simulink model "x2Stage_Rocket"  (R2022b)
settings: Solver=VariableStepAuto  StartTime=0.0  StopTime=5
model workspace: external: MATLAB File C:\Users\Trenton VerKuilen\OneDrive - lmu.edu\School\Capstone\SimscapeImportFiles\x2Stage_Rocket_DataFile.m (data not in the file)
undefined symbols (not defined in the file or in its folder): F, MIL, Moderate, sigbuilder_block, smiData, X, Y, Z
libraries: sm_lib x543, nesl_utility x11, simulink_extras x3, sharedtransform x2, dspmtrx3 x2, aerolibwind2 x2, mspsensorlib x1, aerolibatmos2 x1
(part 11 of 11)

== system x2Stage_Rocket/Model/S1_AvionicsStack_1_RIGID/Stage_2_Electronics_1_RIGID/x2652_BMP280_STEMMA_QT_step_1_RIGID/PCB_Component_step_1_RIGID/x10uF_step_1_RIGID ==
  ReferenceFrame : sm_lib/Frames and Transforms/Reference Frame
  Solid : sm_lib/Body Elements/File Solid  ExtGeomFileName=10uF.step_Default_sldprt.STEP  UnitType=FromFile  ExtGeomFileUnits=m  StepReaderType=HEX  ExportConvexHullGeometry=off  InertiaType=Custom  Mass=smiData.Solid(12).mass  MassUnits=kg  CenterOfMass=smiData.Solid(12).CoM  CenterOfMassUnits=mm  MomentsOfInertia=smiData.Solid(12).MoI  MomentsOfInertiaUnits=kg*mm^2  ProductsOfInertia=smiData.Solid(12).PoI  ProductsOfInertiaUnits=kg*mm^2  BasedOnType=DensityFromFile  Density=1000  DensityUnits=kg/m^3  DoExposeReferenceFrame=on  SerializedFrames=<Frames/>  GraphicType=FromGeometry  MarkerShape=Sphere  MarkerSize=10  GraphicVisPropType=SimpleVisualProperties  GraphicDiffuseColor=smiData.Solid(12).color  GraphicSpecularColor=[0.5 0.5 0.5 1.0]  GraphicAmbientColor=[0.15 0.15 0.15 1.0]  GraphicEmissiveColor=[0.0 0.0 0.0 1.0]  GraphicShininess=75  GraphicOpacity=smiData.Solid(12).opacity
  F : PMIOPort  Side=Left
  connections:
  ReferenceFrame/RConn1 -- Solid/RConn1 -- F/RConn1

== system x2Stage_Rocket/Model/S1_AvionicsStack_1_RIGID/Stage_2_Electronics_1_RIGID/x2652_BMP280_STEMMA_QT_step_1_RIGID/PCB_Component_step_1_RIGID/x10uF_step_2_RIGID ==
  ReferenceFrame : sm_lib/Frames and Transforms/Reference Frame
  Solid : sm_lib/Body Elements/File Solid  ExtGeomFileName=10uF.step_Default_sldprt.STEP  UnitType=FromFile  ExtGeomFileUnits=m  StepReaderType=HEX  ExportConvexHullGeometry=off  InertiaType=Custom  Mass=smiData.Solid(12).mass  MassUnits=kg  CenterOfMass=smiData.Solid(12).CoM  CenterOfMassUnits=mm  MomentsOfInertia=smiData.Solid(12).MoI  MomentsOfInertiaUnits=kg*mm^2  ProductsOfInertia=smiData.Solid(12).PoI  ProductsOfInertiaUnits=kg*mm^2  BasedOnType=DensityFromFile  Density=1000  DensityUnits=kg/m^3  DoExposeReferenceFrame=on  SerializedFrames=<Frames/>  GraphicType=FromGeometry  MarkerShape=Sphere  MarkerSize=10  GraphicVisPropType=SimpleVisualProperties  GraphicDiffuseColor=smiData.Solid(12).color  GraphicSpecularColor=[0.5 0.5 0.5 1.0]  GraphicAmbientColor=[0.15 0.15 0.15 1.0]  GraphicEmissiveColor=[0.0 0.0 0.0 1.0]  GraphicShininess=75  GraphicOpacity=smiData.Solid(12).opacity
  F : PMIOPort  Side=Left
  connections:
  ReferenceFrame/RConn1 -- Solid/RConn1 -- F/RConn1

== system x2Stage_Rocket/Model/S1_AvionicsStack_1_RIGID/Stage_2_Electronics_1_RIGID/x2652_BMP280_STEMMA_QT_step_1_RIGID/PCB_Component_step_1_RIGID/x1N4148_step_1_RIGID ==
  ReferenceFrame : sm_lib/Frames and Transforms/Reference Frame
  Solid : sm_lib/Body Elements/File Solid  ExtGeomFileName=1N4148.step_Default_sldprt.STEP  UnitType=FromFile  ExtGeomFileUnits=m  StepReaderType=HEX  ExportConvexHullGeometry=off  InertiaType=Custom  Mass=smiData.Solid(19).mass  MassUnits=kg  CenterOfMass=smiData.Solid(19).CoM  CenterOfMassUnits=mm  MomentsOfInertia=smiData.Solid(19).MoI  MomentsOfInertiaUnits=kg*mm^2  ProductsOfInertia=smiData.Solid(19).PoI  ProductsOfInertiaUnits=kg*mm^2  BasedOnType=DensityFromFile  Density=1000  DensityUnits=kg/m^3  DoExposeReferenceFrame=on  SerializedFrames=<Frames/>  GraphicType=FromGeometry  MarkerShape=Sphere  MarkerSize=10  GraphicVisPropType=SimpleVisualProperties  GraphicDiffuseColor=smiData.Solid(19).color  GraphicSpecularColor=[0.5 0.5 0.5 1.0]  GraphicAmbientColor=[0.15 0.15 0.15 1.0]  GraphicEmissiveColor=[0.0 0.0 0.0 1.0]  GraphicShininess=75  GraphicOpacity=smiData.Solid(19).opacity
  F : PMIOPort  Side=Left
  connections:
  ReferenceFrame/RConn1 -- Solid/RConn1 -- F/RConn1

== matlab function x2Stage_Rocket/Plant/Aerodynamics/Airframe/Fins Stage 1 ==
  data: C_P_f1 output size=1; C_N_f1 output size=2; C_A_f1 output size=2; AoA input; d_bt input; Re input
function [C_P_f1, C_N_f1, C_A_f1]  = fcn(AoA, d_bt,Re) %only for trapezoidal fins
[C_N_f1, C_P_f1, C_A_f1] = Fins_Stage_1_Coefficients(d_bt, AoA, Re);

== matlab function x2Stage_Rocket/Plant/Overall Rocket/If_on_rail_don't_change ==
  data: Angles input; XYZ_Coords input; Angles_real output; change output
function [Angles_real, change] = fcn(Angles, XYZ_Coords)
[Angles_real, change] = If_on_rail_dont_change(XYZ_Coords, Angles);

== matlab function x2Stage_Rocket/Plant/Overall Rocket/Combine Forces and Convert to Cartesian ==
  data: XYZ_Inertial_Force input; Cart_Accel output; DCM input; Impulse input; Mass input; Inertial_Accel output
function [Cart_Accel,Inertial_Accel]  = fcn(XYZ_Inertial_Force, DCM, Impulse, Mass)
[Cart_Accel,Inertial_Accel] = Combine_Forces_and_Convert_to_Cartesian(XYZ_Inertial_Force, Impulse, Mass, DCM);

== matlab function x2Stage_Rocket/Plant/Aerodynamics/MATLAB Function1 ==
  data: AoA input; Solvable output
function Solvable = fcn(AoA)
if abs(AoA) > deg2rad(15)
    Solvable = 0;
else
    Solvable = 1;
end

== matlab function x2Stage_Rocket/Plant/Aerodynamics/Air Properties/MATLAB Function ==
  settings: updateMethod=CONTINUOUS  sampleTime=0.1
  data: t input; p input; rho output; h input; nu output
function [rho,nu] = AirDensityViscosity(t, p, h)



% AirProperties calculates a variety of air thermodynamic properties from 
% measured values of temperature, pressure and humidity. 
% 
% Variables able to calcuated: 
%   rho         [kg m^-3]       Density
%   mu          [N s m^-2]      Dynamic viscosity
%   k           [W m^-1 K^-1]   Thermal conductivity
%   c_p         [J kg^-1 K^-1]  Specific heat capacity (constant pressure)
%   c_v         [J kg^-1 K^-1]  Specific heat capacity (constant volume)
%   gamma       [1]             Ratio of specific heats
%   c           [m s^-1]        Speed of sound: c = (gamma*R*T/M)^0.5
%   nu          [m^2 s^-1]      Kinematic viscosity: nu = mu/rho
%   alpha       [m^2 s^-1]      Thermal diffusivity: alpha = k/(rho*c_p)
%   Pr          [1]             Prandtl number: Pr = mu*c_p/k
%   M           [kg mol^-1]     Molar mass of humid air
%   R           [J kg^-1 K^-1]  Specific gas constant
%   h           [%]             Relative humidity (if dewpoint inputted)
% 
% Syntax
%   rho = AirProperties
%   [...] = AirProperties(t, p)
%   [...] = AirProperties(t, p, h)
%   [...] = AirProperties(t, p, t_dp, 'DewPoint')
%   [...] = AirProperties(t, p, [], ...)
%   [...] = AirProperties(..., 'xCO2',0.0005)
%   [..., rho]     = AirProperties(..., 'rho')
%   [..., mu]      = AirProperties(..., 'mu')
%   [..., k]       = AirProperties(..., 'k')
%   [..., c_p]     = AirProperties(..., 'c_p')
%   [..., c_v]     = AirProperties(..., 'c_v')
%   [..., gamma]   = AirProperties(..., 'gamma')
%   [..., c]       = AirProperties(..., 'c')
%   [..., nu]      = AirProperties(..., 'nu')
%   [..., alpha]   = AirProperties(..., 'alpha')
%   [..., Pr]      = AirProperties(..., 'Pr')
%   [..., M]       = AirProperties(..., 'M')
%   [..., R]       = AirProperties(..., 'R')
%   [..., h]       = AirProperties(..., 'h')
%   [rho, mu, k, c_p, c_v, gamma, c, nu, alpha, Pr, M, R, h] = AirProperties(t, p, h)
% 
% Inputs
%   <None>      If no inputs are given then it returns the ISA standard air
%               density at 1013.25 hPa and 15°C: 1.225 [kg m^-3].
%               (Recommended value range - see references.)
%   t           ( 15 <= t <= 27  ) [°C]     (m x 1 numeric) Air temperature.
%   p           (600 <= p <= 1100) [hPa]    (m x 1 numeric) Air pressure.
%                   If the pressure is unknown, input [] as p and calculations 
%                   will proceed assuming the standard atmosphere (1013.25 hPa)
%   h           (  0 <= h <= 100 ) [%]      (m x 1 numeric) Relative humidity.
%                   If the humidity is unknown, input [] as h and calculations 
%                   will proceed assuming dry air. 
% 
% Inputs (Optional) 
%   'DewPoint'  Option to calculate the air properties with the dew point rather
%               than the relative humidity. This uses the third input as the 
%               value for dewpoint: t_dp [°C] (t_dp <= t) (m x 1 numeric)
%   'xCO2'      [mol mol^-1] (1 x 1 numeric) Mole fraction of CO2 in the air.
%               Used to improve the estimate of the molar mass of dry air.
%               Default 0.0004.
%   <Output>    (char) The variable to output. 
%               The order of the outputs will follow the input order. 
%               If none of these are provided then the outputs will follow the 
%               default order up to the number of outputs requested (nargout).
%               One or more of the above listed variables. 
% 
% Example Usage
%   rho = AirProperties
%   rho = AirProperties(18)
%   rho = AirProperties(18, 1010)
%   rho = AirProperties(18, 1010, 45)
%   [rho, mu, k] = AirProperties(22, 1010, 18, 'Dewpoint')
%   [rho, mu, k] = AirProperties(18, 1010, 45, 'xCO2', 0.0005)
%   [rho, mu, nu, c] = AirProperties(18, 1010, 45, 'rho', 'mu', 'nu', 'c')
%   [c, nu, mu, rho] = AirProperties(18, 1010, 45, 'c', 'nu', 'mu', 'rho')
%   [c, nu, mu, rho] = AirProperties(18, 1010, [], 'c', 'nu', 'mu', 'rho')
%   [c, nu, mu, rho] = AirProperties(18,   [], [], 'c', 'nu', 'mu', 'rho')
%   
%   t = (15:25)';   p = 1010;           h = 40; 
%   t = 25;         p = (950:10:1040)'; h = 40; 
%   t = 25;         p = 1010;           h = (0:10:100)'; 
%   t = linspace(15,25,10)'; p=linspace(950,1040,10)'; h=linspace(0,100,10)';
%   [rho, mu, k, c, c_p] = AirProperties(t, p, h, 'rho', 'mu', 'k', 'c', 'c_p')
% 
%   t = 0:100; p = 1013.25; h = 0:10:100;
%   n = length(h); Col = repmat((1-1/n:-1/n:0)', 1,3);
%   figure('Position',[50,50,500,400]); hold on; 
%   for ii = 1:n
%       rho(:,ii) = AirProperties(t, [], h(ii), 'rho');
%       plot(t, rho(:,ii), 'color',Col(ii,:));
%   end
%   annotation('textarrow',[0.8,0.75],[0.65,0.35],'String','Humidity')
%   xlabel('Temperature [°C]'); 
%   ylabel('\rho [kg m^{-3}]'); 
%   title('Density of air')
% 
% References:
%   Picard, A, Davis, RS, Glaser, M, Fujii, K, 2008, 'Revised formula for the
%   density of moist air (CIPM-2007)', Metrologia, vol. 45, no. 2, pp. 149-155.
%   DOI: http://dx.doi.org/10.1088/0026-1394/45/2/004
%
%   Tsilingiris, P, 2008, 'Thermophysical and transport properties of humid air
%   at temperature range between 0 and 100°C', Energy Conversion and
%   Management, vol. 49, no. 5, pp.1098-1110. 
%   DOI: https://doi.org/10.1016/j.enconman.2007.09.015
% 
% Shaun Fitzgerald
% Created 2017-09-25
% Modified 
%   2020-03-09  Included calculation of various extra air properties. 
%   2020-11-17  Added to GitHub
%% Inputs 
if nargin == 0
    % ISA standard density of air at 15 °C and 1013.25 hPa
    varout{1} = 1.225;           % [kg m^-3]
    return
end
% Temperature
assert(isnumeric(t) && isvector(t), ...
    'Expected input ''t'' to be a numeric vector or scalar.')
% Pressure
if nargin < 2 || isempty(p)
    p = 1013.25;                    % [hPa] (1 atm)
else
    assert(isnumeric(p) && isvector(p), ...
        'Expected input ''p'' to be a numeric vector or scalar.')
    assert(all(p >= 0), 'Cannot have a negative pressure.')
end
% Humidity
if nargin < 3 || isempty(h)
    UseHumidity = false;
else
    UseHumidity = true;
    assert(isnumeric(h) && isvector(h), ...
        'Expected input ''h'' to be a numeric vector or scalar.')
    assert(all(h >= 0) && all(h <= 100), ...
        'The humidity must be in the range: 0 <= h <= 100.')
end
% Default values
xCO2        = 0.0004;
DewPoint    = false;


%% Basic calculations 
% Constants
R  = 8.314472;                                  % [J mol^-1 K^-1]   Gas Constant
Ma = (28.96546 + 12.011*(xCO2 - 0.0004))*1e-3;  % [kg mol^-1]       Dry air
Mv = 18.01528e-3;                               % [kg mol^-1]       Water Vapour

%% Humidity 
if UseHumidity
    % Saturation vapour pressure
    A =  1.2378847e-5;                          % [K^-2]
    B = -1.9121316e-2;                          % [K^-1]
    C = 33.93711047;                            % [1]
    D = -6.3431645e3;                           % [K]
    p_sv = exp(A*t.^2 + B*t + C + D./t);        % [Pa]
    
    % Enhancement factor
    alpha = 1.00062;                            % [1]
    beta  = 3.14e-8;                            % [Pa^-1]
    gamma = 5.6e-7;                             % [K^-2]
    f = alpha + beta*p + gamma*t.^2;            % [1]
    
    % Mole fraction of water vapour
    if DewPoint    % With dew point temperature
        t_dp = h;
        if any(t_dp > t)
            error('The dew point cannot be greater than the temperature.')
        end
        
        f_dp = alpha + beta*p + gamma*t_dp.^2;  % [1]
        x_v = f_dp.*p_sv./p;                    % [1]
        
        % Calculating relative humidity
        T_dp = t_dp + 273.15;                   % [K]
        p_sv_dp = exp(A*T_dp.^2 + B*T_dp + C + D./T_dp);  % [Pa]
        H = p_sv_dp.*f_dp./(p_sv.*f);           % [1]
        
    else           % With relative humidity
        H = h./100;                             % [1]
        x_v = H.*f.*p_sv./p;                    % [1]
        
    end
    
    % Molar mass of humid air
    M = Ma*(1 - x_v) + Mv*x_v;                  % [kg mol^-1]
    
    % Compressibility Factor
    a0 =  1.58123e-6;                           % [K Pa^-1]
    a1 = -2.93310e-8;                           % [Pa^-1]
    a2 =  1.10430e-10;                          % [K^-1 Pa^-1]
    b0 =  5.70700e-6;                           % [K Pa^-1]
    b1 = -2.05100e-8;                           % [Pa^-1]
    c0 =  1.98980e-4;                           % [K Pa^-1]
    c1 = -2.37600e-6;                           % [Pa^-1]
    d  =  1.83000e-11;                          % [K^2 Pa^-2]
    e  = -0.76500e-8;                           % [K^2 Pa^-2]
    
    Z = 1 - p./t.*(a0 + a1*t + a2*t.^2 + (b0 + b1*t).*x_v + ...
        (c0 + c1*t).*x_v.^2) + p.^2.*t.^-2.*(d + e*x_v.^2);    % [1]
else
    
        OutputNum.h = NaN;
    
    
    % Assuming the molar mass of dry air
    M = Ma;                                     % [kg mol^-1]
    Z = 1;                                      % [1]
end
%% Density & molecular values
rho = p.*M./(R*Z.*t);                           % [kg m^-3]


%% Viscosity 

% Dry air - for 250 <= T <= 600 K
MA0 = -9.8601e-1;
MA1 =  9.080125e-2;
MA2 = -1.17635575e-4;
MA3 =  1.2349703e-7;
MA4 = -5.7971299e-11;
mu_a = (MA0 + MA1*t + MA2*t.^2 + MA3*t.^3 + MA4*t.^4)*1e-6; % [N s m^-2]

if UseHumidity
    % Water vapour - for 0 <= t <= 120 °C
    MV0 = 80.58131868;
    MV1 =  0.4000549451;
    mu_v = (MV0 + MV1*t)*1e-7;              % [N s m^-2]

    % Interaction parameters
    Phi_av = 2^0.5/4*(1+Ma/Mv)^-0.5.*(1+(mu_a./mu_v).^0.5*(Mv/Ma)^0.25).^2;
    Phi_va = 2^0.5/4*(1+Mv/Ma)^-0.5.*(1+(mu_v./mu_a).^0.5*(Ma/Mv)^0.25).^2;

    % Mixture viscosity
    mu = ((1 - x_v).*mu_a)./((1 - x_v) + x_v.*Phi_av) + ...
        (x_v.*mu_v)./(x_v + (1 - x_v).*Phi_va); % [N s m^-2]
else
    mu = mu_a;
end

          % [N s m^-2]


% Kinematic viscosity

nu = mu./rho;                           % [m^2 s^-1]

== matlab function x2Stage_Rocket/Plant/Aerodynamics/Airframe/Body  and Nosecone Coefficients ==
  data: NC_Base_A output; C_P_B output size=1; C_P_NC output size=1; C_N_B output size=2; C_N_NC output size=2; C_A_BN output size=2; L_N input; L_B input; L_C input; D_B input; D_D input; Re input; AoA input; Nu input; K input
function [NC_Base_A,C_P_B,C_P_NC,C_N_B,C_N_NC,C_A_BN] = Coefficients(L_N, L_B, L_C, D_B, D_D, Re, AoA, Nu, K)
[NC_Base_A, C_N_B, C_N_NC, C_A_BN, C_P_NC, C_P_B] = Body_and_Nosecone_Coefficients(Re, L_N, L_B, D_B, D_D, L_C, AoA, Nu, K);

== matlab function x2Stage_Rocket/Plant/Aerodynamics/Airframe/Flaps ==
  data: C_P_flaps output size=1; C_N_flaps output size=2; AoA input; AoA_flaps input; d_bt input; C_A_flaps output size=2; Re input; C_N_roll output size=1
function [C_P_flaps,C_N_flaps,C_A_flaps,C_N_roll] = fcn(AoA,AoA_flaps,d_bt,Re) %only for trapezoidal fins
[C_N_flaps, C_N_roll, C_P_flaps, C_A_flaps] = Active_Fins_Coefficients(d_bt, AoA, AoA_flaps, Re);

== matlab function x2Stage_Rocket/Plant/Aerodynamics/MATLAB Function ==
  data: AoA input; Solvable output
function Solvable = fcn(AoA)
if abs(AoA) > deg2rad(15)
    Solvable = 0;
else
    Solvable = 1;
end

== matlab function x2Stage_Rocket/Plant/Overall Rocket/Calculate AoA and Vel_Magn ==
  data: Wind input; AoA output; Cart_Vel input; Vel_Magn_Rel_Wind output; DCM input; Angles input
function [AoA,Vel_Magn_Rel_Wind] = fcn(Wind, Cart_Vel, DCM, Angles)
[Vel_Magn_Rel_Wind, AoA] = Calculate_AoA_and_Vel_Magn(Wind, Cart_Vel, DCM, Angles);

== matlab function x2Stage_Rocket/Plant/Aerodynamics/Airframe/Fins Stage 2 ==
  data: C_P_f2 output size=1; C_N_f2 output size=2; AoA input; d_bt input; C_A_f2 output size=2; Re input
function [C_P_f2,C_N_f2,C_A_f2] = fcn(AoA, d_bt,Re) %only for trapezoidal fins
[C_N_f2, C_P_f2, C_A_f2] = Fins_Stage_2_Coefficients(d_bt, AoA, Re);
